simulink model "m090_ODE1"  (R2022a)
settings: Solver=VariableStepAuto  StartTime=0.0  StopTime=100  RelTol=1e-3
settings Model: Creator=Admin  LastModifiedBy=Admin

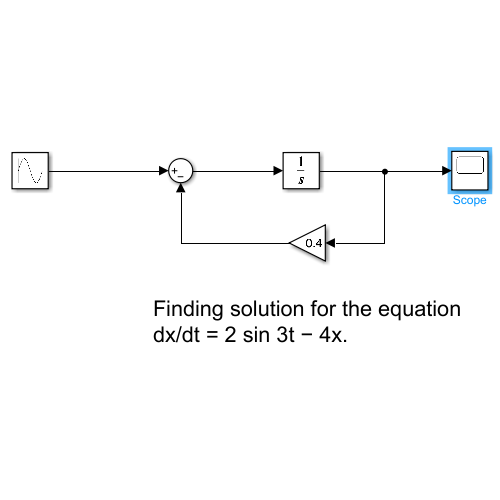
[thumbnail: Simulink's stored preview of the top-level diagram]
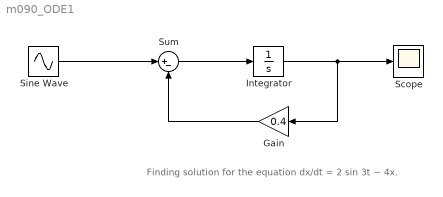
== system m090_ODE1 ==
  note: Finding solution for the equation
      | dx/dt = 2 sin 3t − 4x.
  Gain : Gain  Gain=0.4
  Integrator : Integrator
  Scope : Scope
  Sine Wave : Sin  Amplitude=2  Frequency=3  SampleTime=0
  Sum : Sum  Inputs=|+-
  wires:
  Sine Wave/1 -> Sum/1
  Sum/1 -> Integrator/1
  Integrator/1 -> Gain/1, Scope/1
  Gain/1 -> Sum/2
